simulink library "target_groundpass_lib"  (R2018b)
settings: Solver=VariableStepAuto  StartTime=0.0  StopTime=10.0  RelTol=1e-3
undefined symbols (not defined in the file or in its folder): fswParams
libraries: vrlib x2, simulink x1, sharedutil x1, two_norm x1
settings Model: Creator=taylorreynolds  LastModifiedBy=Taylor

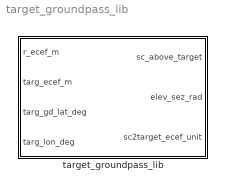
== system target_groundpass_lib ==
  target_groundpass_lib : Subsystem  TreatAsAtomicUnit=on  mask{id=1}
      mask prompts: id "Select the ground target:"
      settings: RTWFcnNameOpts=Use subsystem name  RTWFileNameOpts=Use subsystem name
      mask TypeOptions id: 1 | 2
      mask DialogControl DescGroupVar Prompt: SOC-i Ground Target Selector
      mask DialogControl DescTextVar Prompt: The parameter chosen dictates which ground target the library uses to compute its outputs. The target data are stored in fswParams.ground_target. Target 1 corresponds to the UW groundstation. Target 2 corresponds to the imaging target.

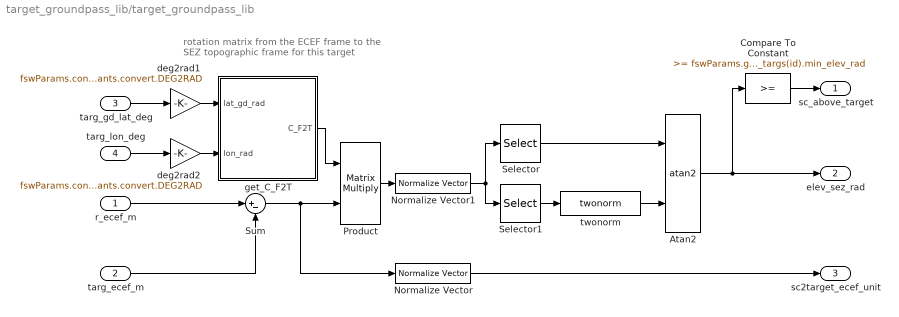
== system target_groundpass_lib/target_groundpass_lib ==
  note: rotation matrix from the ECEF frame to the
      | SEZ topographic frame for this target
  r_ecef_m : Inport
  targ_ecef_m : Inport  Port=2
  targ_gd_lat_deg : Inport  Port=3
  targ_lon_deg : Inport  Port=4
  Atan2 : Trigonometry  Operator=atan2  OutputSignalType=real
  Compare To Constant : simulink/Logic and Bit Operations/Compare To Constant  relop=>=  const=fswParams.ground_targs(id).min_elev_rad  OutDataTypeStr=boolean
  Normalize Vector : vrlib/Utilities/Normalize Vector  maxzero=0
      settings: SourceProductName=Simulink 3D Animation  SourceProductBaseCode=VR
  Normalize Vector1 : vrlib/Utilities/Normalize Vector  maxzero=0
      settings: SourceProductName=Simulink 3D Animation  SourceProductBaseCode=VR
  Product : Product  Multiplication=Matrix(*)
  Selector : Selector  InputPortWidth=3  IndexOptions=Index vector (dialog)  Indices=[3]  OutputSizes=1
  Selector1 : Selector  InputPortWidth=3  IndexOptions=Index vector (dialog)  Indices=[1;2]  OutputSizes=1
  Sum : Sum  Inputs=|+-
  deg2rad1 : Gain  Gain=fswParams.constants.convert.DEG2RAD
  deg2rad2 : Gain  Gain=fswParams.constants.convert.DEG2RAD
  get_C_F2T : Subsystem
  twonorm : two_norm/twonorm  SystemSampleTime=-1
  sc_above_target : Outport
  elev_sez_rad : Outport  Port=2
  sc2target_ecef_unit : Outport  Port=3
  wires:
  r_ecef_m/1 -> Sum/1
  targ_ecef_m/1 -> Sum/2
  Sum/1 -> Normalize Vector/1, Product/2
  Normalize Vector1/1 -> Selector/1, Selector1/1
  Atan2/1 -> Compare To Constant/1, elev_sez_rad/1
  Compare To Constant/1 -> sc_above_target/1
  Normalize Vector/1 -> sc2target_ecef_unit/1
  targ_gd_lat_deg/1 -> deg2rad1/1
  targ_lon_deg/1 -> deg2rad2/1
  get_C_F2T/1(C_F2T) -> Product/1
  deg2rad1/1 -> get_C_F2T/1(lat_gd_rad)
  deg2rad2/1 -> get_C_F2T/2(lon_rad)
  Selector1/1 -> twonorm/1
  twonorm/1 -> Atan2/2
  Selector/1 -> Atan2/1
  Product/1 -> Normalize Vector1/1

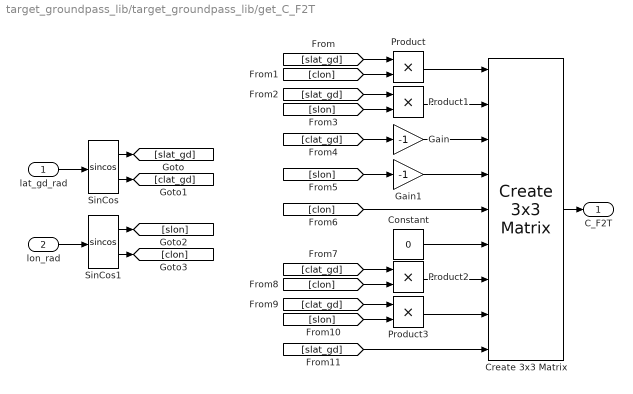
== system target_groundpass_lib/target_groundpass_lib/get_C_F2T ==
  lat_gd_rad : Inport
  lon_rad : Inport  Port=2
  Constant : Constant  Value=0
  Create 3x3 Matrix : sharedutil/Create 3x3 Matrix  aMode=aMode
  Gain : Gain  Gain=-1
  Gain1 : Gain  Gain=-1
  Product{,1..3} (4 alike) : Product
  SinCos : Trigonometry  Operator=sincos  OutputSignalType=real
  SinCos1 : Trigonometry  Operator=sincos  OutputSignalType=real
  C_F2T : Outport
  wires:
  Create 3x3 Matrix/1 -> C_F2T/1
  lat_gd_rad/1 -> SinCos/1
  lon_rad/1 -> SinCos1/1
  Product/1 -> Create 3x3 Matrix/1
  SinCos/1 -> [slat_gd]
  SinCos/2 -> [clat_gd]
  SinCos1/1 -> [slon]
  SinCos1/2 -> [clon]
  [slat_gd] -> Product/1
  [clon] -> Product/2
  Product1/1 -> Create 3x3 Matrix/2
  [slat_gd] -> Product1/1
  [slon] -> Product1/2
  Gain/1 -> Create 3x3 Matrix/3
  [clat_gd] -> Gain/1
  Gain1/1 -> Create 3x3 Matrix/4
  [slon] -> Gain1/1
  [clon] -> Create 3x3 Matrix/5
  Constant/1 -> Create 3x3 Matrix/6
  Product2/1 -> Create 3x3 Matrix/7
  [clat_gd] -> Product2/1
  [clon] -> Product2/2
  Product3/1 -> Create 3x3 Matrix/8
  [clat_gd] -> Product3/1
  [slon] -> Product3/2
  [slat_gd] -> Create 3x3 Matrix/9
